simulink model "Control_schemes_LQR"  (R2022b)
settings: Solver=VariableStepAuto  StartTime=0.0  StopTime=50  RelTol=1e-3
values from neighbouring files (symbols this model uses):
  K_lqr = lqr(sysestc,Q,R)    [Controller.m]    (also in LQR_Controller.m)
undefined symbols (not defined in the file or in its folder): sigbuilder_block
libraries: simulink_extras x7, cstblocks x5, slpidlib x1
settings Model: Creator=AleFire  LastModifiedBy=AleFire

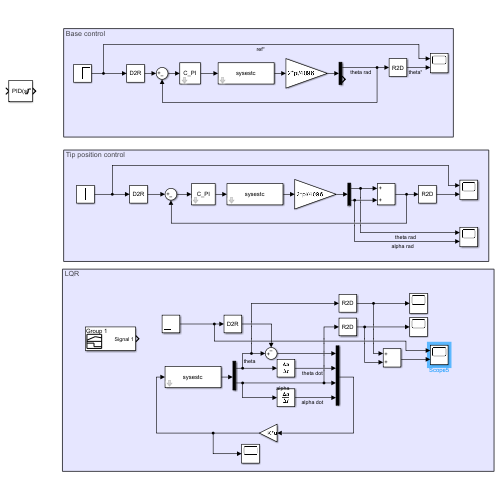
[thumbnail: Simulink's stored preview of the top-level diagram]
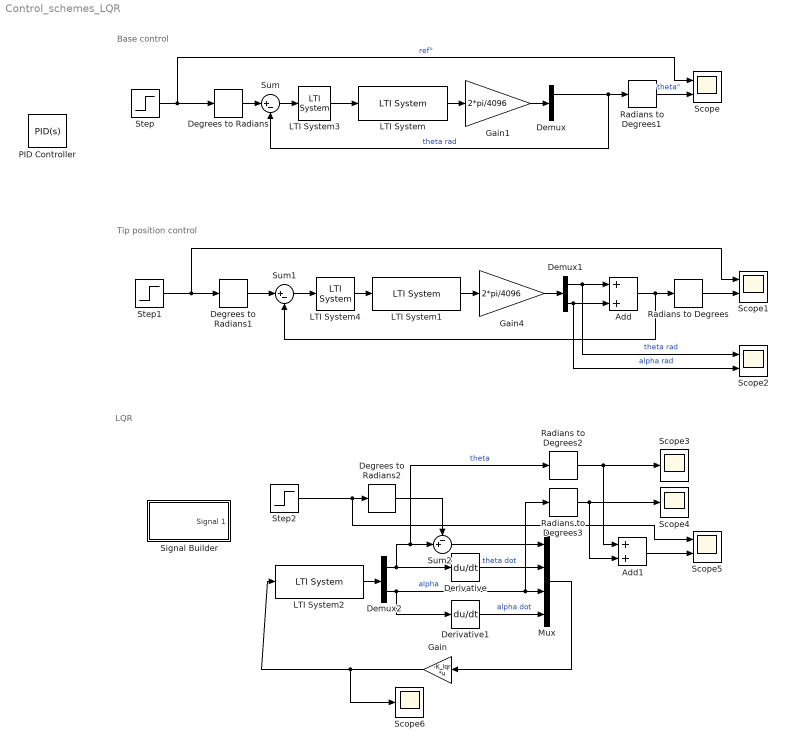
== system Control_schemes_LQR ==
  note: LQR
  note: Tip position control
  note: Base control
  Add : Sum
  Add1 : Sum
  Degrees to Radians : simulink_extras/Transformations/Degrees to Radians
  Degrees to Radians1 : simulink_extras/Transformations/Degrees to Radians
  Degrees to Radians2 : simulink_extras/Transformations/Degrees to Radians
  Demux : Demux  Outputs=2
  Demux1 : Demux  Outputs=2
  Demux2 : Demux  Outputs=2
  Derivative : Derivative
  Derivative1 : Derivative
  Gain : Gain  Gain=-K_lqr  Multiplication=Matrix(K*u)
  Gain1 : Gain  Gain=2*pi/4096
  Gain4 : Gain  Gain=2*pi/4096
  LTI System : cstblocks/LTI System  sys=sysestc  IC=[]
  LTI System1 : cstblocks/LTI System  sys=sysestc  IC=[]
  LTI System2 : cstblocks/LTI System  sys=sysestc  IC=[]
  LTI System3 : cstblocks/LTI System  sys=C_PI  IC=[]
  LTI System4 : cstblocks/LTI System  sys=C_PI  IC=[]
  Mux : Mux
  PID Controller : slpidlib/PID Controller  Controller=PID  Form=Parallel  TimeDomain=Continuous-time  UseExternalTs=off  SampleTime=-1  IntegratorMethod=Forward Euler  FilterMethod=Forward Euler  ControllerParametersSource=internal  P=500  I=100  UseKiTs=off  D=100  N=3.68188133779263  UseFilter=on  TunerSelectOption=Transfer Function Based (PID Tuner App)  InitialConditionSource=internal  InitialConditionForIntegrator=0  InitialConditionForFilter=0  DifferentiatorICPrevScaledInput=0  ExternalReset=none  TrackingMode=off  Kt=1  LimitOutput=on  SatLimitsSource=internal  UpperSaturationLimit=4.5  LowerSaturationLimit=-4.5  LinearizeAsGain=on  AntiWindupMode=clamping  Kb=1  LimitIntegrator=off  UpperIntegratorSaturationLimit=inf  LowerIntegratorSaturationLimit=-inf  POutMin=[]  POutMax=[]  IOutMin=[]  IOutMax=[]  DOutMin=[]  DOutMax=[]  NOutMin=[]  NOutMax=[]  SumOutMin=[]  SumOutMax=[]  SaturationOutMin=[]  SaturationOutMax=[]  PParamMin=[]  PParamMax=[]  IParamMin=[]  IParamMax=[]  DParamMin=[]  DParamMax=[]  NParamMin=[]  NParamMax=[]  KbParamMin=[]  KbParamMax=[]  KtParamMin=[]  KtParamMax=[]  KbOutMin=[]  KbOutMax=[]  KtOutMin=[]  KtOutMax=[]  IntegratorOutMin=[]  IntegratorOutMax=[]  FilterOutMin=[]  FilterOutMax=[]  SumI1OutMin=[]  SumI1OutMax=[]  SumI2OutMin=[]  SumI2OutMax=[]  SumI3OutMin=[]  SumI3OutMax=[]  SumI4OutMin=[]  SumI4OutMax=[]  SumDOutMin=[]  SumDOutMax=[]  DifferentiatorOutMin=[]  DifferentiatorOutMax=[]  FilterDiffOutCoefMin=[]  FilterDiffOutCoefMax=[]  ReciprocalOutMin=[]  ReciprocalOutMax=[]  SumDenOutMin=[]  SumDenOutMax=[]  SumNumOutMin=[]  SumNumOutMax=[]  DivideOutMin=[]  DivideOutMax=[]  UdiffTsProdOutMin=[]  UdiffTsProdOutMax=[]  NTsProdOutMin=[]  NTsProdOutMax=[]  UintegralTsProdOutMin=[]  UintegralTsProdOutMax=[]  UngainTsProdOutMin=[]  UngainTsProdOutMax=[]  ClampingZeroOutDataTypeStr=Inherit: Inherit via back propagation  ClampingZeroOutMin=[]  ClampingZeroOutMax=[]  FilterDenConstantOutDataTypeStr=Inherit: Inherit via back propagation  FilterDenConstantOutMin=[]  FilterDenConstantOutMax=[]  PCopyOutDataTypeStr=Inherit: Inherit via back propagation  PCopyOutMin=[]  PCopyOutMax=[]  NCopyOutDataTypeStr=Inherit: Inherit via back propagation  NCopyOutMin=[]  NCopyOutMax=[]  IntegratorContinuousStateAttributes=''  IntegratorStateMustResolveToSignalObject=off  IntegratorRTWStateStorageClass=Auto  FilterContinuousStateAttributes=''  FilterStateMustResolveToSignalObject=off  FilterRTWStateStorageClass=Auto  ParallelPVariant=InternalParameters  IdealPVariant=Disabled  IVariant=InternalParameters  DVariant=InternalParameters  IntegratorVariant=Continuous  SatVariant=Enabled  AWVariant=ContClampingParallel  PCopyVariant=Disabled  TRVariant=Disabled  FdbkBlocksVariant=Forward  IdealPFdbkVariant=Disabled  SatFdbkVariant=Disabled  DerivativeFilterVariant=ContFilter  NVariant=InternalParameters  NCopyVariant=Disabled  FilterICVariant=InternalICsFilter  IntegratorICVariant=InternalICs  ExternalResetVariant=Disabled  TRSumVariant=Passthrough  SumFdbkVariant=Disabled  SumVariant=Sum_PID  TsampFilterVariant=InternalTs  TsampNgainVariant=Passthrough  TsampIntegralVariant=Passthrough  ExternalSaturationOutDataTypeStr=Inherit: Same as second input
  Radians to Degrees{,1..3} (4 alike) : simulink_extras/Transformations/Radians to Degrees
  Scope{,1..2,5} (4 alike) : Scope  NumInputPorts=2
  Scope3 : Scope
  Scope4 : Scope
  Scope6 : Scope
  Signal Builder : Subsystem  Tag=STV Subsys  LoadFcn=sigbuilder_block('load');  StartFcn=sigbuilder_block('start');  StopFcn=sigbuilder_block('stop');  ClipboardFcn=sigbuilder_block('clipboard');  mask(Sigbuilder block){tuvar=[0:10]}
      mask help: Simulink:masks:SigbuilderBlock_MD
      mask init:
      | if ~strcmp(get_param(bdroot(gcbh),'SimulationStatus'),'stopped') tuvar = sigbuilder_block('maskInit'); end
      settings: CopyFcn=sigbuilder_block('copy');  DeleteFcn=sigbuilder_block('delete');  ModelCloseFcn=sigbuilder_block('modelClose');  PreSaveFcn=sigbuilder_block('preSave');  PauseFcn=sigbuilder_block('pause');  ContinueFcn=sigbuilder_block('continue');  NameChangeFcn=sigbuilder_block('namechange');  OpenFcn=sigbuilder_block('open',[437.6 199.2 550.4 400 ]);  CloseFcn=sigbuilder_block('close');
      mask Display: plot(0, 0, 100, 100,[2, 2, 32, 32, 2], [68, 8, 8, 68, 68],[32, 2], [38, 38], [32, 19, 2],[53, 60, 44], [32, 17, 17, 2],[16, 16, 31, 31]);txt = getActiveGroup(gcbh);text(2, 100, txt,'verticalAlignment', 'top');
  Step : Step  After=20  SampleTime=0
  Step1 : Step  After=20  SampleTime=0
  Step2 : Step  Time=5  After=20  SampleTime=0
  Sum : Sum  Inputs=|+-
  Sum1 : Sum  Inputs=|+-
  Sum2 : Sum  Inputs=-+|
  wires:
  Step/1 -> Degrees to Radians/1, Scope/1  "ref°"
  Degrees to Radians/1 -> Sum/1
  Demux/1 -> Radians to Degrees1/1, Sum/2  "theta rad"
  LTI System/1 -> Gain1/1
  Gain1/1 -> Demux/1
  Radians to Degrees1/1 -> Scope/2  "theta°"
  LTI System1/1 -> Gain4/1
  Radians to Degrees/1 -> Scope1/2
  Add/1 -> Radians to Degrees/1, Sum1/2
  Gain4/1 -> Demux1/1
  Degrees to Radians1/1 -> Sum1/1
  Step1/1 -> Degrees to Radians1/1, Scope1/1
  Demux1/1 -> Scope2/1, Add/1  "theta rad"
  Demux1/2 -> Scope2/2, Add/2  "alpha rad"
  Degrees to Radians2/1 -> Sum2/1
  LTI System2/1 -> Demux2/1
  Demux2/1 -> Radians to Degrees2/1, Sum2/2, Derivative/1  "theta"
  Derivative/1 -> Mux/2  "theta dot"
  Mux/1 -> Gain/1
  Demux2/2 -> Derivative1/1, Radians to Degrees3/1, Mux/3  "alpha"
  Derivative1/1 -> Mux/4  "alpha dot"
  Gain/1 -> Scope6/1, LTI System2/1
  Sum2/1 -> Mux/1
  Radians to Degrees2/1 -> Add1/1, Scope3/1
  Radians to Degrees3/1 -> Add1/2, Scope4/1
  Add1/1 -> Scope5/2
  Step2/1 -> Scope5/1, Degrees to Radians2/1
  Sum1/1 -> LTI System4/1
  LTI System4/1 -> LTI System1/1
  Sum/1 -> LTI System3/1
  LTI System3/1 -> LTI System/1

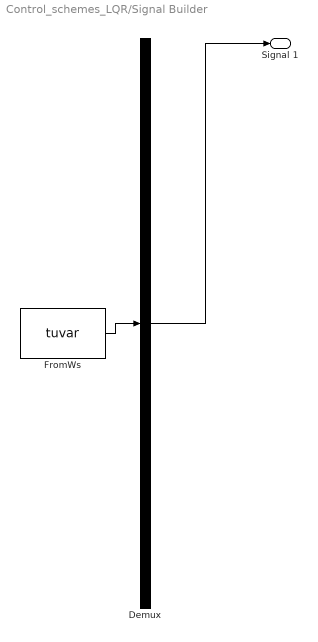
== system Control_schemes_LQR/Signal Builder ==
  Demux : Demux  Tag=STV Demux  Outputs=1
      settings: DisplayOption=none
  FromWs : FromWorkspace  Tag=STV FromWs  VariableName=tuvar
      SigBuilderData=|
      | common.afterFinalStr = 'Extrapolate'
      | common.sampleTime = 0
      | dataSet.timeRange = [0 10]
      | dataSet.name = 'Group 1'
      | sbobj.Groups.Name = 'Group 1'
      | sbobj.Groups.Signals.Name = 'Signal 1'
      | sbobj.Groups.Signals.XData = [0 0.94 2 2 2.82 4 4 6 6 7.6 10]
      | sbobj.Groups.Signals.YData = [0 1.015 1.01 -0.285 0.83 0.125 0.665 0.785 -0.24 -0.325 0]
  Signal 1 : Outport  Tag=STV Outport
  wires:
  Demux/1 -> Signal 1/1
  FromWs/1 -> Demux/1
